simulink model "Assembly_union"  (R2020a)
settings: Solver=VariableStepAuto  StartTime=0.0  StopTime=inf  RelTol=1e-3
model workspace: external: MATLAB File A:\Usuarios\TATTO PC\Desktop\univesidad\Procesamiento video y audio\proyecto 6 intelingencia artificial\Assembly3_DataFile.m (data not in the file)
undefined symbols (not defined in the file or in its folder): smiData, X, Y, Z
libraries: neural x563, sm_lib x153, nesl_utility x4, dspstat3 x3, audiosources x1, simulink x1, dspxfrm3 x1
(part 36 of 36)

== matlab function Assembly_union/MATLAB Function ==
  data: x output; u input; y output; v input; c output; ang input; signo input
function [x,y,c]= fcn(u,v,ang,signo)


if v>u 
    if v>1 && v<3
        %y=2;
        c=0
        if (ang<0.1) || (6.27<ang && ang<6.29) || (12.4<ang && ang<12.6)
        y=0.1;
        x=0;
        elseif (1.56<ang && ang<1.58) || (7.7<ang && ang<7.9) || (14<ang && ang<14.2)
        y=0;
        x=-0.1*signo;
        elseif (3.13<ang && ang<3.15) || (9.3<ang && ang<9.5) || (15.6<ang && ang<15.8)
        y=-0.1;
        x=0;
        elseif (4.70<ang && ang<4.72) || (10.9<ang && ang<11) || (17.2<ang && ang<17.4)
        y=0;
        x=0.1*signo;
        else
            x=0;
            y=0;
        end 
    elseif v>3 && v<5
       % y=4;
        c=1.57
        y=0;
        x=0;
    elseif v>5 && v<7
       % y=6;
       c=-1.57
       y=0;
       x=0;
    elseif v>7
       % y=8;
        c=0
        if (ang<0.1) || (6.27<ang && ang<6.29) || (12.4<ang && ang<12.6)
        y=-0.1;
        x=0;
        elseif (1.56<ang && ang<1.58) || (7.7<ang && ang<7.9) || (14<ang && ang<14.2)
        y=0;
        x=0.1*signo;
        elseif (3.13<ang && ang<3.15) || (9.3<ang && ang<9.5) || (15.6<ang && ang<15.8)
        y=0.1;
        x=0;
        elseif (4.70<ang && ang<4.72) || (10.9<ang && ang<11) || (17.2<ang && ang<17.4)
        y=0;
        x=-0.1*signo;
        else
            x=0;
            y=0;
        end
    else
        y=0;
        x=0;
        c=0
    end
    
else
    y=0;
    x=0;
    c=0;
end

== matlab function Assembly_union/Subsystem/FFTSHIFT ==
  data: u input; y output
function y = fcn(u)
x=abs(u(8:1024/2-442));
x1=max(x);
if x1 >=0.03
y = x
else
    y = zeros(63,1)
end
